simulink model "Topic3"  (R2015a)
settings: Solver=ode45  StartTime=0.0  StopTime=10.0  RelTol=1e-3
libraries: roblocks x3, simulink x1
settings Model: Creator=Alexander Liao  LastModifiedBy=Alexander Liao

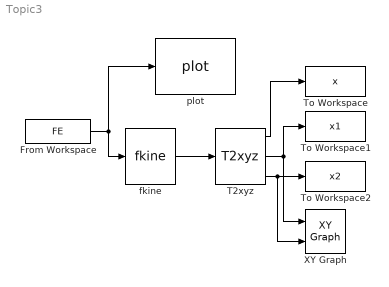
== system Topic3 ==
  From Workspace : FromWorkspace  VariableName=FE  OutputAfterFinalValue=Holding final value
  T2xyz : roblocks/Transform Conversion/T2xyz
  To Workspace : ToWorkspace  VariableName=x  SampleTime=-1
      settings: Save2DSignal=2-D array (concatenate along first dimension)
  To Workspace1 : ToWorkspace  VariableName=x1  SampleTime=-1
      settings: Save2DSignal=2-D array (concatenate along first dimension)
  To Workspace2 : ToWorkspace  VariableName=x2  SampleTime=-1
      settings: Save2DSignal=2-D array (concatenate along first dimension)
  XY Graph : simulink/Sinks/XY Graph  xmin=-1  xmax=1  ymin=-1  ymax=1  st=-1
  fkine : roblocks/Kinematics/fkine  robot=p560
  plot : roblocks/Robot Graphics/plot  robot=p560  fps=25  holdplot=on
  wires:
  fkine/1 -> T2xyz/1
  T2xyz/3 -> XY Graph/2, To Workspace2/1
  T2xyz/1 -> To Workspace/1
  T2xyz/2 -> XY Graph/1, To Workspace1/1
  From Workspace/1 -> fkine/1, plot/1
